simulink model "first_model"  (R2018b)
settings: Solver=VariableStepAuto  StartTime=0.0  StopTime=10.0  RelTol=1e-3
settings Model: Creator=mikoto  LastModifiedBy=mikoto

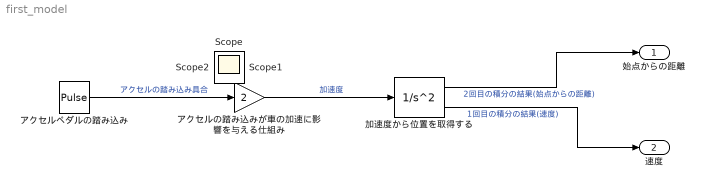
== system first_model ==
  アクセルの踏み込みが車の加速に影響を与える仕組み : Gain  Gain=2
  "アクセルペダルの踏み込み " : DiscretePulseGenerator  PulseType=Time based  Period=10  PulseWidth=5
  加速度から位置を取得する : SecondOrderIntegrator  ICX=0
  始点からの距離 : Outport
  速度 : Outport  Port=2
  Scope : Scope
  Scope1 : Scope
  Scope2 : Scope
  wires:
  "アクセルペダルの踏み込み "/1 -> アクセルの踏み込みが車の加速に影響を与える仕組み/1  "アクセルの踏み込み具合"
  アクセルの踏み込みが車の加速に影響を与える仕組み/1 -> 加速度から位置を取得する/1  "加速度"
  加速度から位置を取得する/1 -> 始点からの距離/1  "2回目の積分の結果(始点からの距離)"
  加速度から位置を取得する/2 -> 速度/1  "1回目の積分の結果(速度)"
